simulink model "simulation"  (R2021b)
settings: Solver=VariableStepAuto  StartTime=0.0  StopTime=10  MaxStep=0.001  MinStep=0.0001  RelTol=1e-3
libraries: fl_lib x9, nesl_utility x5
settings Model: Creator=Roberto  LastModifiedBy=Roberto

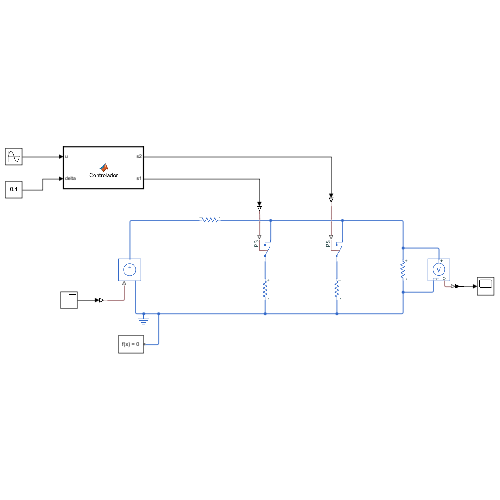
[thumbnail: Simulink's stored preview of the top-level diagram]
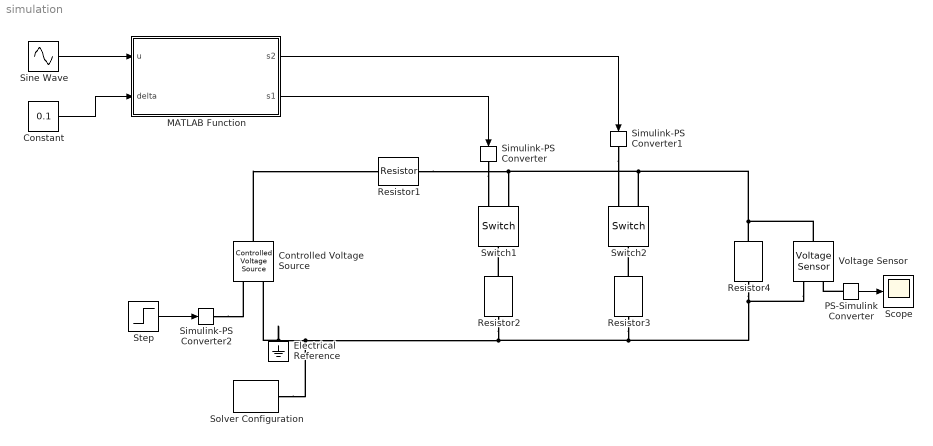
== system simulation ==
  Constant : Constant  Value=0.1
  Controlled Voltage Source : fl_lib/Electrical/Electrical Sources/Controlled Voltage Source
  Electrical Reference : fl_lib/Electrical/Electrical Elements/Electrical Reference
  MATLAB Function : MATLAB Function  TreatAsAtomicUnit=on
  PS-Simulink Converter : nesl_utility/PS-Simulink Converter  PhysicalDomain=network_engine_domain  SubClassName=ps_output  LeftPortType=input  RightPortType=output  PseudoPeriodic=off  Frequencies=[]  Unit=inherit  AffineConversion=off
      settings: SourceProductBaseCode=PW,SS
  Resistor{1..4} (4 alike) : fl_lib/Electrical/Electrical Elements/Resistor  R=1 Ohm  i_specify=off  i_priority=None  i=0 A  i_nominal_specify=off  i_nominal_unit=A  i_nominal_value=1  v_specify=off  v_priority=None  v=0 V  v_nominal_specify=off  v_nominal_unit=V  v_nominal_value=1
  Scope : Scope
  Simulink-PS Converter : nesl_utility/Simulink-PS Converter  PhysicalDomain=network_engine_domain  SubClassName=ps_input  LeftPortType=input  RightPortType=output  PseudoPeriodic=off  Frequencies=[]  NoiseDistribution=none  NoiseParameters=[]  Unit=1  AffineConversion=off  FilteringAndDerivatives=provide  SimscapeFilterOrder=1  InputFilterTimeConstant=0.001  UdotUserProvided=0
      settings: SourceProductBaseCode=PW,SS
  Simulink-PS Converter1 : nesl_utility/Simulink-PS Converter  PhysicalDomain=network_engine_domain  SubClassName=ps_input  LeftPortType=input  RightPortType=output  PseudoPeriodic=off  Frequencies=[]  NoiseDistribution=none  NoiseParameters=[]  Unit=1  AffineConversion=off  FilteringAndDerivatives=provide  SimscapeFilterOrder=1  InputFilterTimeConstant=0.001  UdotUserProvided=0
      settings: SourceProductBaseCode=PW,SS
  Simulink-PS Converter2 : nesl_utility/Simulink-PS Converter  PhysicalDomain=network_engine_domain  SubClassName=ps_input  LeftPortType=input  RightPortType=output  PseudoPeriodic=off  Frequencies=[]  NoiseDistribution=none  NoiseParameters=[]  Unit=1  AffineConversion=off  FilteringAndDerivatives=provide  SimscapeFilterOrder=1  InputFilterTimeConstant=0.001  UdotUserProvided=0
      settings: SourceProductBaseCode=PW,SS
  Sine Wave : Sin  Amplitude=10  Frequency=5  SampleTime=0
  Solver Configuration : nesl_utility/Solver Configuration  PhysicalDomain=network_engine_domain  SubClassName=solver  LeftPortType=input  RightPortType=generic  Tones=[]  Harmonics=[]  SimulateNoise=off  Profile=off  UseLocalSampling=off  EnableSwitchedLinearOptims=on  FrequencyDomain=off  UseCCode=off  RelTol=0.001  AbsTol=1e-06  MinStep=1e-09  ToWorkspace=off  RevertToSquareIcSolve=off  NumHomotopyIterations=100  PhasorMode=off  PhasorModeNumHarmonics=1  DoDC=off  ResidualTolerance=1e-09  UseLocalSolver=off  LocalSolverChoice=NE_BACKWARD_EULER_ADVANCER  LocalSolverSampleTime=0.001  DoFixedCost=off  MaxNonlinIter=3  MaxModeIter=2  ComputeImpulses=off  ImpulseIterations=2  LinearAlgebra=auto  EquationFormulation=NE_TIME_EF  DelaysMemoryBudget=1024  AutomaticFiltering=on  FilteringTimeConstant=0.001  PartitionStorageMethod=AS_NEEDED  PartitionMemoryBudget=1024  PartitionMethod=ROBUST
      settings: SourceProductBaseCode=PW,SS
  Step : Step  SampleTime=0
  Switch1 : fl_lib/Electrical/Electrical Elements/Switch  R_closed=0.01 Ohm  G_open=1e-8 1/Ohm  Threshold=0.5  i_specify=off  i_priority=None  i=0 A  i_nominal_specify=off  i_nominal_unit=A  i_nominal_value=1  v_specify=off  v_priority=None  v=0 V  v_nominal_specify=off  v_nominal_unit=V  v_nominal_value=1
  Switch2 : fl_lib/Electrical/Electrical Elements/Switch  R_closed=0.01 Ohm  G_open=1e-8 1/Ohm  Threshold=0.5  i_specify=off  i_priority=None  i=0 A  i_nominal_specify=off  i_nominal_unit=A  i_nominal_value=1  v_specify=off  v_priority=None  v=0 V  v_nominal_specify=off  v_nominal_unit=V  v_nominal_value=1
  Voltage Sensor : fl_lib/Electrical/Electrical Sensors/Voltage Sensor
  wires:
  Sine Wave/1 -> MATLAB Function/1(u)
  Step/1 -> Simulink-PS Converter2/1
  PS-Simulink Converter/1 -> Scope/1
  MATLAB Function/2(s1) -> Simulink-PS Converter/1
  MATLAB Function/1(s2) -> Simulink-PS Converter1/1
  Constant/1 -> MATLAB Function/2(delta)
  connections:
  Controlled Voltage Source/LConn1 -- Resistor1/LConn1
  Resistor1/RConn1 -- Voltage Sensor/LConn1 -- Resistor4/LConn1 -- Switch2/RConn2 -- Switch1/RConn2
  Resistor3/LConn1 -- Switch2/LConn1
  Resistor2/LConn1 -- Switch1/LConn1
  Resistor4/RConn1 -- Voltage Sensor/RConn2 -- Resistor3/RConn1 -- Solver Configuration/RConn1 -- Controlled Voltage Source/RConn2 -- Electrical Reference/LConn1 -- Resistor2/RConn1
  Simulink-PS Converter2/RConn1 -- Controlled Voltage Source/RConn1
  PS-Simulink Converter/LConn1 -- Voltage Sensor/RConn1
  Simulink-PS Converter/RConn1 -- Switch1/RConn1
  Simulink-PS Converter1/RConn1 -- Switch2/RConn1

== matlab function simulation/MATLAB Function ==
  data: s2 output; u input; s1 output; delta input
function [s2, s1] = Controlador(u,delta)


        if u < -delta
            theta_1 = 0;
            theta_2 = pi/2;
           
        elseif ( u >= -delta) && (u < 0)
            theta_1 = (pi/2)*((u/delta)+1);
            theta_2 = -(pi/2)*(u/delta);   
            
        elseif u == 0
            theta_1 = pi/2;
            theta_2 = 0;
            
        elseif (u > 0) && (u <= delta)
            theta_1 = (pi/2)*(-(u/delta)+1);
            theta_2 = (pi/2)*(u/delta); 
            
        elseif u > delta
            theta_1 = 0;
            theta_2 = pi/2;
            
        else
            theta_1 = 0;
            theta_2 = pi/2;           
        end

            p1 = (cos(theta_1)*cos(theta_2))^2;
            p2 = (cos(theta_1)*sin(theta_1))^2;
            p3 = (sin(theta_1)*cos(theta_2))^2;
            p4 = (sin(theta_1)*sin(theta_2))^2;
    
        if p1 > 0.5
            s1 = 0;
            s2 = 0;
        elseif p2 > 0.5
            s1 = 1;
            s2 = 0;
        elseif p3 > 0.5
            s1 = 0;
            s2 = 1;
        elseif p4 > 0.5
            s1 = 1;
            s2 = 1;
        else
            s1 = 1;
            s2 = 1;
        end
end
